simulink model "exaktlin"  (Simulink 10.1)
settings: Solver=ode45  StartTime=0.0  StopTime=10.0  RelTol=1e-3  EnableMultiTasking=on
values from neighbouring files (symbols this model uses):
  L = place(A, B, [-2, -2.3])    [lab3.m]    (also in lab3_prepp.m = place(A, B, [-30, -40]))
  Lr = pinv( dcgain( Gc_no_feedforward ) )    [lab3.m]    (also in lab3_prepp.m = pinv(dcgain(Gc_no_feedforward)))
settings Model: Creator=axelsson  LastModifiedBy=David Wiman
settings DataIOCC: LimitDataPoints=on  SignalLoggingSaveFormat=ModelDataLogs
settings OptimizationCC: ExpressionDepthLimit=2147483647
settings DebuggingCC: SolverPrmCheckMsg=warning  FcnCallInpInsideContextMsg=warning  StateNameClashWarn=warning

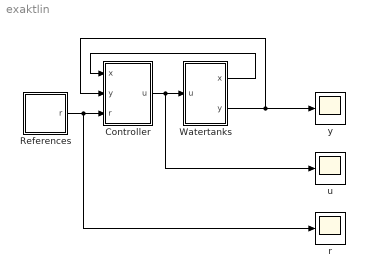
== system exaktlin ==
  Controller : Subsystem
  References : Subsystem  mask{t1=5, r0=5, r1=1}
      mask prompts: t1 "Tid för steget"; r0 "Startnivå"; r1 "Höjd på steget"
  Watertanks : Subsystem
  r : Scope
  u : Scope
  y : Scope
  wires:
  Controller/1(u) -> u/1, Watertanks/1(u)
  References/1(r) -> Controller/3(r), r/1
  Watertanks/1(x) -> Controller/1(x)
  Watertanks/2(y) -> Controller/2(y), y/1

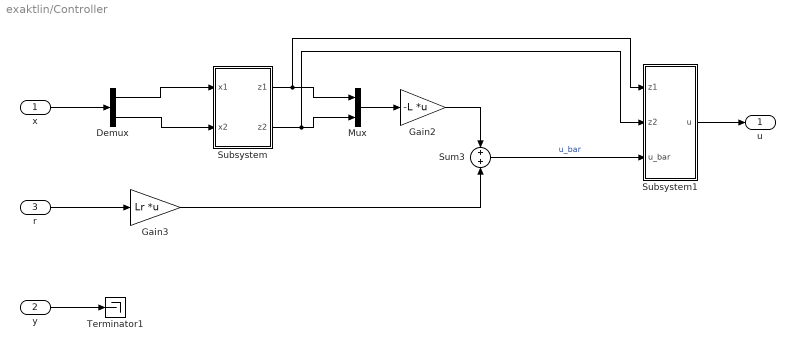
== system exaktlin/Controller ==
  x : Inport
  y : Inport  Port=2
  r : Inport  Port=3
  Demux : Demux  Outputs=2
  Gain2 : Gain  Gain=-L  Multiplication=Matrix(K*u)
  Gain3 : Gain  Gain=Lr  Multiplication=Matrix(K*u)
  Mux : Mux  Inputs=2
  Subsystem : Subsystem
  Subsystem1 : Subsystem
  Sum3 : Sum  Inputs=+|+
  Terminator1 : Terminator
  u : Outport
  wires:
  x/1 -> Demux/1
  y/1 -> Terminator1/1
  Subsystem1/1(u) -> u/1
  Demux/1 -> Subsystem/1(x1)
  Demux/2 -> Subsystem/2(x2)
  Subsystem/1(z1) -> Mux/1, Subsystem1/1(z1)
  Subsystem/2(z2) -> Subsystem1/2(z2), Mux/2
  Mux/1 -> Gain2/1
  Gain2/1 -> Sum3/1
  r/1 -> Gain3/1
  Gain3/1 -> Sum3/2
  Sum3/1 -> Subsystem1/3(u_bar)  "u_bar"

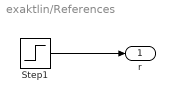
== system exaktlin/References ==
  Step1 : Step  Time=t1  Before=r0  After=r0+r1  SampleTime=0
  r : Outport
  wires:
  Step1/1 -> r/1

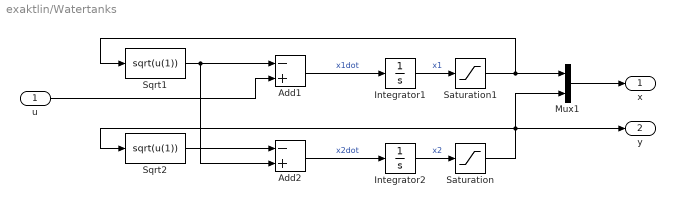
== system exaktlin/Watertanks ==
  u : Inport
  Add1 : Sum  Inputs=-+
  Add2 : Sum  Inputs=-+
  Integrator1 : Integrator  InitialCondition=5
  Integrator2 : Integrator  InitialCondition=5
  Mux1 : Mux  Inputs=2
  Saturation : Saturate  UpperLimit=100  LowerLimit=0
  Saturation1 : Saturate  UpperLimit=100  LowerLimit=0
  Sqrt1 : Fcn  Expr=sqrt(u(1))
  Sqrt2 : Fcn  Expr=sqrt(u(1))
  x : Outport
  y : Outport  Port=2
  wires:
  Integrator1/1 -> Saturation1/1  "x1"
  Integrator2/1 -> Saturation/1  "x2"
  Sqrt2/1 -> Add2/1
  Add2/1 -> Integrator2/1  "x2dot"
  Sqrt1/1 -> Add2/2, Add1/1
  Add1/1 -> Integrator1/1  "x1dot"
  u/1 -> Add1/2
  Mux1/1 -> x/1
  Saturation/1 -> Sqrt2/1, y/1, Mux1/2
  Saturation1/1 -> Sqrt1/1, Mux1/1

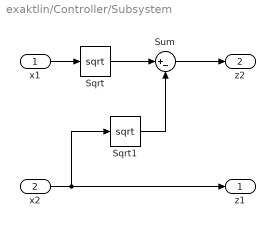
== system exaktlin/Controller/Subsystem ==
  x1 : Inport
  x2 : Inport  Port=2
  Sqrt : Sqrt  SaturateOnIntegerOverflow=on
  Sqrt1 : Sqrt  SaturateOnIntegerOverflow=on
  Sum : Sum  Inputs=|+-
  z1 : Outport
  z2 : Outport  Port=2
  wires:
  x2/1 -> Sqrt1/1, z1/1
  x1/1 -> Sqrt/1
  Sqrt/1 -> Sum/1
  Sqrt1/1 -> Sum/2
  Sum/1 -> z2/1

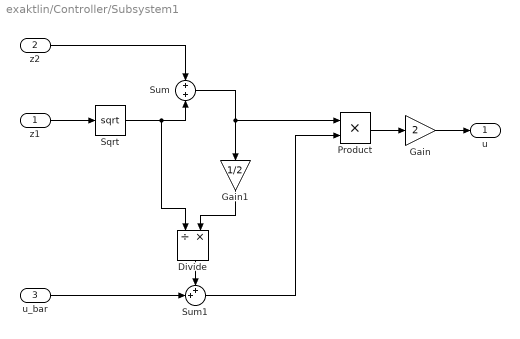
== system exaktlin/Controller/Subsystem1 ==
  z1 : Inport
  z2 : Inport  Port=2
  u_bar : Inport  Port=3
  Divide : Product  Inputs=/*
  Gain : Gain  Gain=2
  Gain1 : Gain  Gain=1/2
  Product : Product
  Sqrt : Sqrt  SaturateOnIntegerOverflow=on
  Sum : Sum  Inputs=+|+
  Sum1 : Sum  Inputs=++|
  u : Outport
  wires:
  Sum/1 -> Product/1, Gain1/1
  Product/1 -> Gain/1
  Sum1/1 -> Product/2
  z1/1 -> Sqrt/1
  Gain/1 -> u/1
  z2/1 -> Sum/1
  Sqrt/1 -> Sum/2, Divide/1
  Gain1/1 -> Divide/2
  u_bar/1 -> Sum1/2
  Divide/1 -> Sum1/1
